simulink model "SERIE"  (R2023a)
settings: Solver=VariableStepAuto  StartTime=0.0  StopTime=2/Frequency  RelTol=1e-3
undefined symbols (not defined in the file): C, Frequency, L, R, V
libraries: spsFourierLib x4, spsSeriesRLCBranchLib x3, spsMultimeterLib x1, spsACVoltageSourceLib x1, sps_lib x1
settings Model: Creator=XIOMARA  LastModifiedBy=XIOMARA

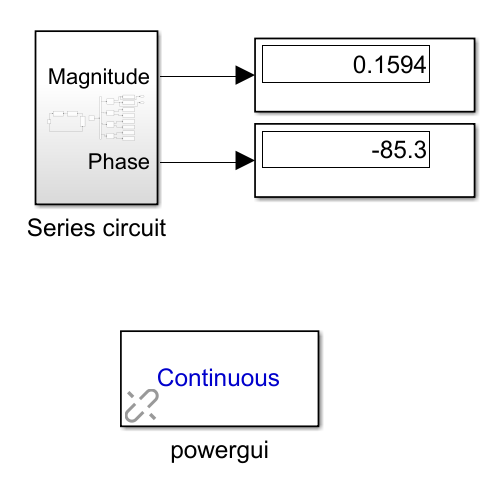
[thumbnail: Simulink's stored preview of the top-level diagram]
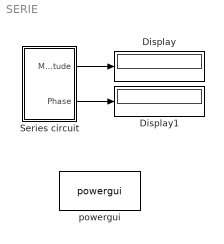
== system SERIE ==
  Display : Display
  Display1 : Display
  Series circuit : Subsystem
  powergui : sps_lib/powergui  Priority=1  SimulationMode=Continuous  SampleTime=50e-6  frequency=60  Iterations=50  frequencyindice=1000000  Pbase=100e6  ErrMax=1e-4  UnitsV=kV  UnitsW=MW  buscounter=0  FunctionMessages=off  echomessages=off  EnableUseOfTLC=off  CurrentSourceSwitches=off  DisableSnubberDevices=off  DisableRonSwitches=off  DisableVfSwitches=off  DisplayEquations=off  AutomaticDiscreteSolvers=off  SolverType=Tustin/Backward Euler (TBE)  Interpol=off  ExternalGateDelay=off  methode=off  Ts=100  x0status=blocks  SPID=on  SwTol=0  HookPort=off  NonlinearTolerance=1e-4  nMaxIteration=100  ContinueOnMaxIteration=off  RestoreLinks=warning  ResistiveCurrentMeasurement=off  Frange=[0:2:500]  Ylog=off  Xlog=on  ShowGrid=off  save=off  variable=ZData  structure=0  ZoomFFT=off  StartTime=0.0  cycles=1  DisplayStyle=1  fundamental=60  FreqAxis=off  MaxFrequency=1000  frequencyindicesteady=1  RmsSteady=1  display=off
  wires:
  Series circuit/1(Magnitude) -> Display/1
  Series circuit/2(Phase) -> Display1/1

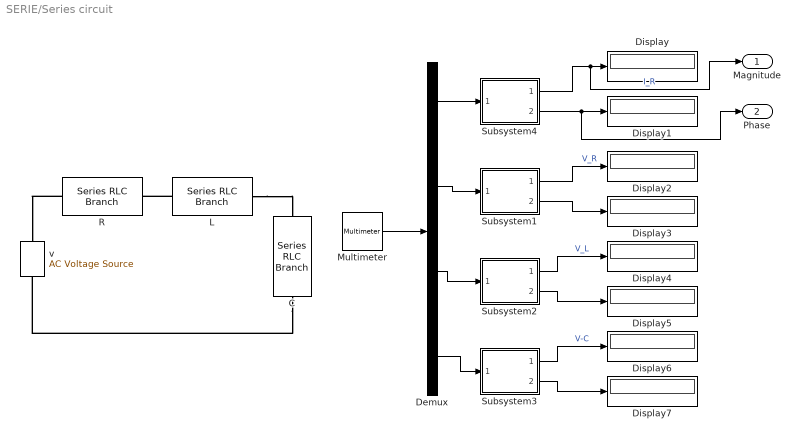
== system SERIE/Series circuit ==
  "C " : spsSeriesRLCBranchLib/Series RLC Branch  LConnTagsString=__new0  RConnTagsString=__new0  BranchType=C  Resistance=1  Inductance=1e-3  SetiL0=off  InitialCurrent=0  Capacitance=C  Setx0=off  InitialVoltage=0  Measurements=Branch voltage
  Demux : Demux
  Display{,1..7} (8 alike) : Display
  L : spsSeriesRLCBranchLib/Series RLC Branch  LConnTagsString=__new0  RConnTagsString=__new0  BranchType=L  Resistance=1  Inductance=L  SetiL0=off  InitialCurrent=0  Capacitance=1e-6  Setx0=off  InitialVoltage=0  Measurements=Branch voltage
  Multimeter : spsMultimeterLib/Multimeter  L=4  sel=[4 3 2 1]  yselected={}  Gain=[1 1 1 1]  OutputType=Complex  PlotAtSimulationStop=off  PhasorSimulation=off
  R : spsSeriesRLCBranchLib/Series RLC Branch  LConnTagsString=__new0  RConnTagsString=__new0  BranchType=R  Resistance=R  Inductance=1e-3  SetiL0=off  InitialCurrent=0  Capacitance=1e-6  Setx0=off  InitialVoltage=0  Measurements=Branch voltage and current
  Subsystem1 : Subsystem
  Subsystem2 : Subsystem
  Subsystem3 : Subsystem
  Subsystem4 : Subsystem
  v : spsACVoltageSourceLib/AC Voltage Source  Amplitude=V*sqrt(2)  Phase=0  Frequency=Frequency  SampleTime=0  Measurements=None  BusType=swing  Pref=10e3  Qref=0  Qmin=-inf  Qmax=+inf
  Magnitude : Outport
  Phase : Outport  Port=2
  wires:
  Subsystem2/1(Magnitude) -> Display4/1  "V_L"
  Subsystem1/1(Magnitude) -> Display2/1  "V_R"
  Demux/2 -> Subsystem1/1(Signal)
  Subsystem2/2(Phase) -> Display5/1
  Subsystem3/1(Magnitude) -> Display6/1  "V-C"
  Demux/1 -> Subsystem4/1(Signal)
  Subsystem1/2(Phase) -> Display3/1
  Demux/4 -> Subsystem3/1(Signal)
  Demux/3 -> Subsystem2/1(Signal)
  Subsystem3/2(Phase) -> Display7/1
  Subsystem4/1(Magnitude) -> Magnitude/1, Display/1  "I_R"
  Subsystem4/2(Phase) -> Phase/1, Display1/1
  Multimeter/1 -> Demux/1
  connections:
  R/LConn1 -- v/RConn1
  "C "/RConn1 -- v/LConn1
  L/RConn1 -- "C "/LConn1
  L/LConn1 -- R/RConn1

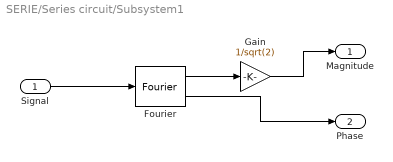
== system SERIE/Series circuit/Subsystem1 ==
  Signal : Inport
  Fourier : spsFourierLib/Fourier  Freq=Frequency  n=1  InInit=[0, 0]  Ts=0
  Gain : Gain  Gain=1/sqrt(2)
  Magnitude : Outport
  Phase : Outport  Port=2
  wires:
  Fourier/1 -> Gain/1
  Gain/1 -> Magnitude/1
  Signal/1 -> Fourier/1
  Fourier/2 -> Phase/1

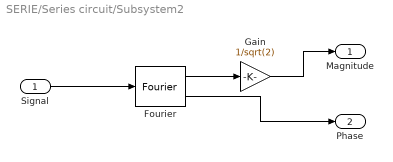
== system SERIE/Series circuit/Subsystem2 ==
  Signal : Inport
  Fourier : spsFourierLib/Fourier  Freq=Frequency  n=1  InInit=[0, 0]  Ts=0
  Gain : Gain  Gain=1/sqrt(2)
  Magnitude : Outport
  Phase : Outport  Port=2
  wires:
  Fourier/1 -> Gain/1
  Gain/1 -> Magnitude/1
  Signal/1 -> Fourier/1
  Fourier/2 -> Phase/1

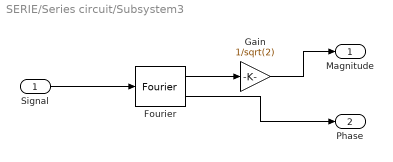
== system SERIE/Series circuit/Subsystem3 ==
  Signal : Inport
  Fourier : spsFourierLib/Fourier  Freq=Frequency  n=1  InInit=[0, 0]  Ts=0
  Gain : Gain  Gain=1/sqrt(2)
  Magnitude : Outport
  Phase : Outport  Port=2
  wires:
  Fourier/1 -> Gain/1
  Gain/1 -> Magnitude/1
  Signal/1 -> Fourier/1
  Fourier/2 -> Phase/1

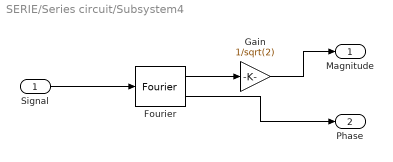
== system SERIE/Series circuit/Subsystem4 ==
  Signal : Inport
  Fourier : spsFourierLib/Fourier  Freq=Frequency  n=1  InInit=[0, 0]  Ts=0
  Gain : Gain  Gain=1/sqrt(2)
  Magnitude : Outport
  Phase : Outport  Port=2
  wires:
  Fourier/1 -> Gain/1
  Gain/1 -> Magnitude/1
  Signal/1 -> Fourier/1
  Fourier/2 -> Phase/1
